simulink model "Fuel_Pump_V3_1_20201113_20KHz"  (R2019b)
settings: configuration reference "Configuration" (kept outside this file)
PreLoadFcn:
  | RTWConfigurationCB('preloadfcn', bdroot);
values from neighbouring files (symbols this model uses):
  MotorPara_Base_Frq = 666.0    [fuel_pump_V3_1_20201113_20kHz.sldd]
  MotorPara_Base_I = 50.0    [fuel_pump_V3_1_20201113_20kHz.sldd]
  MotorPara_Base_RPM = 12000.0    [fuel_pump_V3_1_20201113_20kHz.sldd]
  MotorPara_Base_V = 28.0    [fuel_pump_V3_1_20201113_20kHz.sldd]
  MotorPara_Ld = 1.287E-5    [fuel_pump_V3_1_20201113_20kHz.sldd]
  MotorPara_Lq = 2.052E-5    [fuel_pump_V3_1_20201113_20kHz.sldd]
  MotorPara_Ls = 8.3475E-5    [fuel_pump_V3_1_20201113_20kHz.sldd]
  MotorPara_P = 4.0    [fuel_pump_V3_1_20201113_20kHz.sldd]
  MotorPara_Rs = 0.01638    [fuel_pump_V3_1_20201113_20kHz.sldd]
  TPBRD_HALF = 1875.0    [fuel_pump_V3_1_20201113_20kHz.sldd]
  Ts_1kHz = 0.001    [fuel_pump_V3_1_20201113_20kHz.sldd]
  Ts_200Hz = 0.005    [fuel_pump_V3_1_20201113_20kHz.sldd]
  Ts_20KHz = 5.0E-5    [fuel_pump_V3_1_20201113_20kHz.sldd]
  Ts_40Hz = 0.025    [fuel_pump_V3_1_20201113_20kHz.sldd]
  Ts_50Hz = 0.02    [fuel_pump_V3_1_20201113_20kHz.sldd]
undefined symbols (not defined in the file or in its folder): DiscIntNeverNeededParam, Down, Up
libraries: c280xlib x22, c2833xlib x6, c2837xDlib x4, c28xdmclib x4, etargetslib x4, dspstat3 x2, c2000lib x1, idelinklib_common x1
(part 2 of 4)

== system Fuel_Pump_V3_1_20201113_20KHz/SCI_TX ==
  1-D Lookup Table2 : Lookup_n-D  Commented=on  NumberOfTableDimensions=1  BreakpointsForDimension1=[0,9.84,53.12,85.06,128.14,168.25,208.63,249.25,290.69,331.14,368.31]  Table=[0,-1000,-2000,-3000,-4000,-5000,-6000,-7000,-8000,-9000,-10000]  InternalRulePriority=Speed  RndMeth=Simplest  InputSameDT=on
  Data Store Read13 : DataStoreRead  Commented=on  DataStoreName=WFm
  Data Store Write : DataStoreWrite  Commented=on  DataStoreName=nDem
  FPM : Subsystem
  MATLAB Function49 : MATLAB Function  Commented=on  TreatAsAtomicUnit=on
  SCI Receive2 : c280xlib/SCI Receive  Commented=on  sciModule=A  dataHead='~~'  dataTail=''  dataType=uint8  dataDim=10  initValue=0  errOption=Output custom value  errValue=[255,0,0,0,0,0,0,0,0,255]  sampleTime=Ts_SCI  outputStatus=off  postInterrupt=off  numFifo=10
      settings: SourceProductName=Embedded Coder Support Package for Texas Instruments C2000 Processors  SourceProductBaseCode=TIC2000
  SCI Transmit : c280xlib/SCI Transmit  sciModule=A  dataHead=''  dataTail=''  postInterrupt=off  numFifo=1
      settings: SourceProductName=Embedded Coder Support Package for Texas Instruments C2000 Processors
  SCI_TX : Subsystem
  Saturation : Saturate  Commented=on  UpperLimit=0  LowerLimit=-12000
  wires:
  Data Store Read13/1 -> 1-D Lookup Table2/1
  1-D Lookup Table2/1 -> Saturation/1
  Saturation/1 -> Data Store Write/1
  SCI Receive2/1 -> MATLAB Function49/1(Data_SCI)
  SCI_TX/1(SCI_DATA) -> SCI Transmit/1

== system Fuel_Pump_V3_1_20201113_20KHz/Set_nDem ==
  Data Store Read1 : DataStoreRead  DataStoreName=n_Step
  Data Store Read2 : DataStoreRead  DataStoreName=nDem
  Data Store Read3 : DataStoreRead  Commented=on  DataStoreName=LWF_Step
  Data Store Read4 : DataStoreRead  Commented=on  DataStoreName=LWFDem
  Data Store Write1 : DataStoreWrite  DataStoreName=nDem_PI
  Data Store Write2 : DataStoreWrite  Commented=on  DataStoreName=Set_Speed
  Data Store Write3 : DataStoreWrite  Commented=on  DataStoreName=SMO_KP
  Data Store Write4 : DataStoreWrite  Commented=on  DataStoreName=SMO_KI
  Data Store Write5 : DataStoreWrite  DataStoreName=SMO_Filter
  Gain : Gain  Gain=1/MotorPara_Base_RPM
  Gain1 : Gain  Gain=MotorPara_Base_RPM
  Gain2 : Gain  Commented=on  Gain=13/3  OutDataTypeStr=Inherit: Inherit via back propagation
  Gain3 : Gain  Commented=on  Gain=15000  OutDataTypeStr=Inherit: Inherit via back propagation
  Gain4 : Gain  Commented=on  Gain=5*2*pi/60*4
  Gain5 : Gain  Commented=on  Gain=2
  Gain6 : Gain  Gain=10
  Gain7 : Gain  Gain=-1
  MATLAB Function1 : MATLAB Function  TreatAsAtomicUnit=on
  MATLAB Function2 : MATLAB Function  Commented=on  TreatAsAtomicUnit=on
  Square : Math  Commented=on  Operator=square  SignedPower=off  SaturateOnIntegerOverflow=on
  wires:
  Data Store Read2/1 -> Gain/1
  MATLAB Function1/1(Set_Point) -> Gain1/1
  Data Store Read1/1 -> MATLAB Function1/2(Step)
  Data Store Read4/1 -> Gain2/1
  Data Store Read3/1 -> MATLAB Function2/2(Step)
  Gain3/1 -> Data Store Write2/1
  Gain2/1 -> MATLAB Function2/1(Target)
  MATLAB Function2/1(Set_Point) -> Gain3/1
  Gain/1 -> MATLAB Function1/1(Target)
  Gain1/1 -> Gain7/1, Data Store Write1/1
  Gain4/1 -> Square/1, Gain5/1
  Gain5/1 -> Data Store Write3/1
  Square/1 -> Data Store Write4/1
  Gain6/1 -> Data Store Write5/1
  Gain7/1 -> Gain6/1, Gain4/1

== system Fuel_Pump_V3_1_20201113_20KHz/System Initialize ==

== system Fuel_Pump_V3_1_20201113_20KHz/IIC_Interrupt /Subsystem ==
  function : TriggerPort  TriggerType=function-call  VariantControl=Variant
  Data Store Write2 : DataStoreWrite  DataStoreName=TEMP_MOT1
  Demux : Demux  Outputs=2
  I2C Receive : c280xlib/I2C Receive  Priority=1  selectModule=I2C_A  addrFormat=7-Bit addressing  saSource=Specify via dialog  SAR=64  bitCount=8  dataLength=2  initValue=0  NACK=off  STP=on  STR=off  sampleTime=-1  dataType=uint8
      settings: SourceProductName=Embedded Coder Support Package for Texas Instruments C2000 Processors  SourceProductBaseCode=TIC2000
  Temp_conv : MATLAB Function  TreatAsAtomicUnit=on
  wires:
  Temp_conv/1(y) -> Data Store Write2/1
  I2C Receive/1 -> Demux/1
  Demux/2 -> Temp_conv/2(u2)
  Demux/1 -> Temp_conv/1(u1)

== system Fuel_Pump_V3_1_20201113_20KHz/IIC_Interrupt /Subsystem1 ==
  function : TriggerPort  TriggerType=function-call  VariantControl=Variant
  Data Store Write2 : DataStoreWrite  DataStoreName=TEMP_MOT2
  Demux : Demux  Outputs=2
  I2C Receive : c280xlib/I2C Receive  Priority=1  selectModule=I2C_A  addrFormat=7-Bit addressing  saSource=Specify via dialog  SAR=65  bitCount=8  dataLength=2  initValue=0  NACK=off  STP=on  STR=off  sampleTime=-1  dataType=uint8
      settings: SourceProductName=Embedded Coder Support Package for Texas Instruments C2000 Processors  SourceProductBaseCode=TIC2000
  Temp_conv : MATLAB Function  TreatAsAtomicUnit=on
  wires:
  Demux/1 -> Temp_conv/1(u1)
  Demux/2 -> Temp_conv/2(u2)
  I2C Receive/1 -> Demux/1
  Temp_conv/1(y) -> Data Store Write2/1

== system Fuel_Pump_V3_1_20201113_20KHz/IIC_PT1000/Subsystem4 ==
  function : TriggerPort  TriggerType=function-call  VariantControl=Variant
  Constant : Constant  Value=16  OutDataTypeStr=uint8  SampleTime=-1
  I2C Transmit : c280xlib/I2C Transmit  selectModule=I2C_A  addrFormat=7-Bit addressing  saSource=Specify via dialog  SAR=64  bitCount=8  STP=off  RM=off  STR=off
      settings: SourceProductName=Embedded Coder Support Package for Texas Instruments C2000 Processors  SourceProductBaseCode=TIC2000
  wires:
  Constant/1 -> I2C Transmit/1

== system Fuel_Pump_V3_1_20201113_20KHz/IIC_PT1000/Subsystem5 ==
  function : TriggerPort  TriggerType=function-call  VariantControl=Variant
  Constant : Constant  Value=16  OutDataTypeStr=uint8  SampleTime=-1
  I2C Transmit : c280xlib/I2C Transmit  selectModule=I2C_A  addrFormat=7-Bit addressing  saSource=Specify via dialog  SAR=65  bitCount=8  STP=off  RM=off  STR=off
      settings: SourceProductName=Embedded Coder Support Package for Texas Instruments C2000 Processors  SourceProductBaseCode=TIC2000
  wires:
  Constant/1 -> I2C Transmit/1

== system Fuel_Pump_V3_1_20201113_20KHz/Motor_Control/Initial Case ==
  Action Port : ActionPort  ActionPortLabel=case [ 0 ]:

== system Fuel_Pump_V3_1_20201113_20KHz/Motor_Control/Interrupt_Count ==
  Add : Sum
  Constant : Constant  OutDataTypeStr=uint16  SampleTime=-1
  Constant1 : Constant  Value=0.00005  OutDataTypeStr=single  SampleTime=-1
  Product : Product  OutDataTypeStr=uint8
  Saturation : Saturate  UpperLimit=40000  LowerLimit=0
  Unit Delay : UnitDelay  SampleTime=-1  HasFrameUpgradeWarning=on
  Out1 : Outport
  wires:
  Product/1 -> Out1/1
  Unit Delay/1 -> Add/2
  Add/1 -> Saturation/1
  Saturation/1 -> Product/2, Unit Delay/1
  Constant1/1 -> Product/1
  Constant/1 -> Add/1

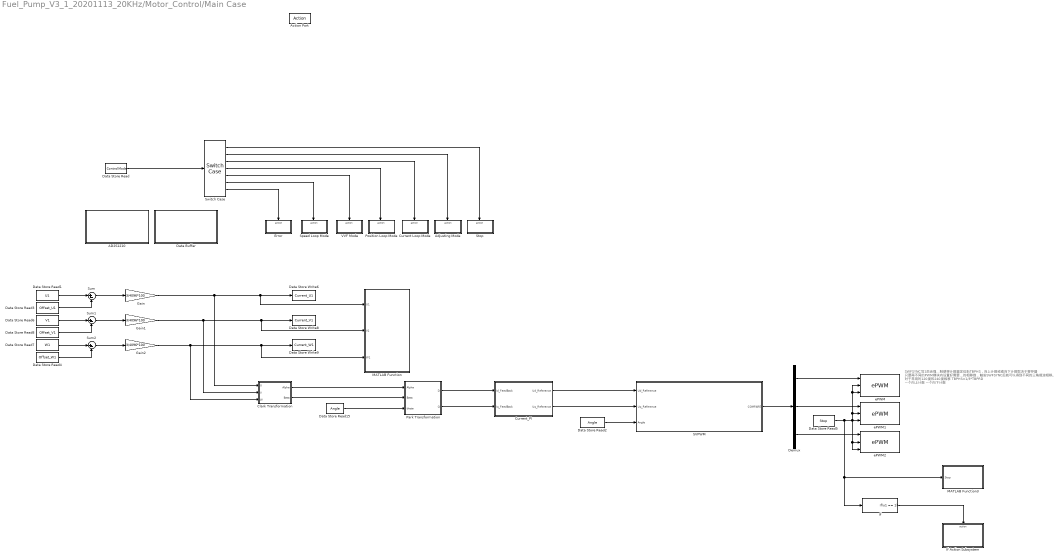
== system Fuel_Pump_V3_1_20201113_20KHz/Motor_Control/Main Case  ==
  note: SWFSYNC写1后会强制使得计数器定位到TBPHS，向上计数或者向下计数取决于寄存器
      |
      | 只要再不同的PWM模块内设置好需要的相移数，触发SWFSYNC后就可以得到不同的三角载波相移。
      |
      | 对于常用的120度和240度相移
      | TBPHS=1/3*TBPRD 一个向上计数 一个向下计数
  Action Port : ActionPort  ActionPortLabel=case [ 2 ]:
  AD2S1210 : Subsystem  Priority=30  TreatAsAtomicUnit=on
  Adjusting Mode : Subsystem  TreatAsAtomicUnit=on
  Clark Transformation : Subsystem
  Current Loop Mode : Subsystem  TreatAsAtomicUnit=on
  Current_PI : Subsystem  TreatAsAtomicUnit=on
      settings: RTWSystemCode=Inline
  "Data Buffer " : Subsystem
  Data Store Read : DataStoreRead  Priority=40  DataStoreName=ControlMode
  Data Store Read1 : DataStoreRead  DataStoreName=U1
  Data Store Read15 : DataStoreRead  Priority=62  DataStoreName=Angle
  Data Store Read2 : DataStoreRead  DataStoreName=Angle
  Data Store Read3 : DataStoreRead  DataStoreName=Offset_U1
  Data Store Read4 : DataStoreRead  DataStoreName=Offset_W1
  Data Store Read5 : DataStoreRead  DataStoreName=Stop
  Data Store Read6 : DataStoreRead  DataStoreName=V1
  Data Store Read7 : DataStoreRead  DataStoreName=W1
  Data Store Read8 : DataStoreRead  DataStoreName=Offset_V1
  Data Store Write6 : DataStoreWrite  DataStoreName=Current_U1
  Data Store Write8 : DataStoreWrite  DataStoreName=Current_V1
  Data Store Write9 : DataStoreWrite  DataStoreName=Current_W1
  Demux : Demux  Outputs=3
  Error : Subsystem  TreatAsAtomicUnit=on
  Gain : Gain  Gain=3/4096*100  OutDataTypeStr=single
  Gain1 : Gain  Gain=3/4096*100  OutDataTypeStr=single
  Gain2 : Gain  Gain=3/4096*100  OutDataTypeStr=single
  If : If  IfExpression=u1 == 1  ShowElse=off
  If Action Subsystem : Subsystem  TreatAsAtomicUnit=on
  MATLAB Function : MATLAB Function  TreatAsAtomicUnit=on
  MATLAB Function3 : MATLAB Function  TreatAsAtomicUnit=on
  Park Transformation : Subsystem
  Position Loop Mode : Subsystem  TreatAsAtomicUnit=on
  SVPWM : Subsystem  TreatAsAtomicUnit=on
      settings: RTWSystemCode=Inline
  Speed Loop Mode : Subsystem  TreatAsAtomicUnit=on
  Stop : Subsystem  TreatAsAtomicUnit=on
  Sum : Sum  Inputs=|+-  AccumDataTypeStr=int16  OutDataTypeStr=int16  InputSameDT=on
  Sum1 : Sum  Inputs=|+-  AccumDataTypeStr=int16  OutDataTypeStr=int16  InputSameDT=on
  Sum2 : Sum  Inputs=|+-  AccumDataTypeStr=int16  OutDataTypeStr=int16  InputSameDT=on
  Switch Case : SwitchCase  CaseConditions={0,1,2,3,4,5}
  VVF Mode : Subsystem  TreatAsAtomicUnit=on
  ePWM : c280xlib/ePWM  checkMode=off  useModule=ePWM1  periodUnits=Clock cycles  timerSource=Specify via dialog  timerPeriod_clk=TPBRD  timerPeriod_sec=0.0001  tbshadow=Counter equals to zero  countingMode=Up-Down  phaseActiveEnable=Set counter to phase value specified via dialog  phaseDirection=Count down after sync  phaseActive=0  synchronizationEnable=off  synchronizationOption=Counter equals to zero (CTR=Zero)  clockPrescale=1  HSclockPrescale=1  ePWMxAStatus=on  CMPAUnits=Clock cycles  CMPASource=Input port  CMPAValue_per=50  CMPAValue_clk=0  enCMPAshadow=Counter equals to zero  ePWMxAactionLogic1=Do nothing  ePWMxAactionLogic2=Do nothing  ePWMxAactionLogic3=Set  ePWMxAactionLogic4=Clear  ePWMxAactionLogic5=Do nothing  ePWMxAactionLogic6=Do nothing  ePWMxALoadMode=Load on counter equals to zero (CTR=Zero)  ePWMxACSFenable=on  ePWMxACSFvalue=Forcing disable  ePWMxASFreload=Immediate  enHRPWM=off  HRPWM_LoadMode=Counter equals to zero (CTR=ZERO)  HRPWM_CTLMode=Phase control mode  HRPWM_EDGMode=Both edge  enSFO=on  ePWMxBStatus=on  CMPBUnits=Clock cycles  CMPBSource=Specify via dialog  CMPBValue_per=50  CMPBValue_clk=0  enCMPBshadow=Counter equals to zero  ePWMxBactionLogic1=Do nothing  ePWMxBactionLogic2=Do nothing  ePWMxBactionLogic3=Set  ePWMxBactionLogic4=Clear  ePWMxBactionLogic5=Do nothing  ePWMxBactionLogic6=Do nothing  ePWMxBLoadMode=Load on counter equals to zero (CTR=Zero)  ePWMxBCSFenable=on  ePWMxBCSFvalue=Forcing disable  ePWMxBSFreload=Immediate  enableDBePWMxA=on  enableDBePWMxB=on  DBpolarity=Active high (AH)  DBedgeDelay=Negative  DBSource_ePWMxA=ePWMxA  DBSource_ePWMxB=ePWMxA  DBperiodSource=Specify via dialog  REDperiod=TDEAD  FEDperiod=TDEAD  adcstartModuleA=on  adcrequestEventA=First event  adcstartEventA=Counter equals to zero (CTR=Zero)  adcstartModuleB=off  adcrequestEventB=First event  adcstartEventB=Counter equals to zero (CTR=Zero)  intEn=off  intPrd=First event  intSel=Counter equals to zero (CTR=Zero)  chopperEnable=off  chopperFrequency=1  chopperFirstwidth=1  chopperDuty=12.5%  tripZonesource=Specify via dialog  tzselOSHT1=off  tzselOSHT2=off  tzselOSHT3=off  tzselOSHT4=off  tzselOSHT5=off  tzselOSHT6=off  tzselCBC1=off  tzselCBC2=off  tzselCBC3=off  tzselCBC4=off  tzselCBC5=off  tzselCBC6=off  enTzOstIntr=off  enTzCbcIntr=off  ePWMxAforced=No action  ePWMxBforced=No action  timerPeriod=-1  ePWMxAValue=0  ePWMxBValue=0  tripZoneoption=One-shot trip (OSHT)
      settings: SourceProductName=Embedded Coder Support Package for Texas Instruments C2000 Processors  SourceProductBaseCode=TIC2000
  ePWM1 : c280xlib/ePWM  checkMode=off  useModule=ePWM2  periodUnits=Clock cycles  timerSource=Specify via dialog  timerPeriod_clk=TPBRD  timerPeriod_sec=0.0001  tbshadow=Counter equals to zero  countingMode=Up-Down  phaseActiveEnable=Set counter to phase value specified via dialog  phaseDirection=Count down after sync  phaseActive=0  synchronizationEnable=off  synchronizationOption=Counter equals to zero (CTR=Zero)  clockPrescale=1  HSclockPrescale=1  ePWMxAStatus=on  CMPAUnits=Clock cycles  CMPASource=Input port  CMPAValue_per=50  CMPAValue_clk=0  enCMPAshadow=Counter equals to zero  ePWMxAactionLogic1=Do nothing  ePWMxAactionLogic2=Do nothing  ePWMxAactionLogic3=Set  ePWMxAactionLogic4=Clear  ePWMxAactionLogic5=Do nothing  ePWMxAactionLogic6=Do nothing  ePWMxALoadMode=Load on counter equals to zero (CTR=Zero)  ePWMxACSFenable=on  ePWMxACSFvalue=Forcing disable  ePWMxASFreload=Immediate  enHRPWM=off  HRPWM_LoadMode=Counter equals to zero (CTR=ZERO)  HRPWM_CTLMode=Phase control mode  HRPWM_EDGMode=Both edge  enSFO=on  ePWMxBStatus=on  CMPBUnits=Clock cycles  CMPBSource=Specify via dialog  CMPBValue_per=50  CMPBValue_clk=0  enCMPBshadow=Counter equals to zero  ePWMxBactionLogic1=Do nothing  ePWMxBactionLogic2=Do nothing  ePWMxBactionLogic3=Set  ePWMxBactionLogic4=Clear  ePWMxBactionLogic5=Do nothing  ePWMxBactionLogic6=Do nothing  ePWMxBLoadMode=Load on counter equals to zero (CTR=Zero)  ePWMxBCSFenable=on  ePWMxBCSFvalue=Forcing disable  ePWMxBSFreload=Immediate  enableDBePWMxA=on  enableDBePWMxB=on  DBpolarity=Active high (AH)  DBedgeDelay=Positive  DBSource_ePWMxA=ePWMxA  DBSource_ePWMxB=ePWMxA  DBperiodSource=Specify via dialog  REDperiod=TDEAD  FEDperiod=TDEAD  adcstartModuleA=off  adcrequestEventA=First event  adcstartEventA=Counter equals to period (CTR=PRD)  adcstartModuleB=off  adcrequestEventB=First event  adcstartEventB=Counter equals to zero (CTR=Zero)  intEn=off  intPrd=First event  intSel=Counter equals to zero (CTR=Zero)  chopperEnable=off  chopperFrequency=1  chopperFirstwidth=1  chopperDuty=12.5%  tripZonesource=Specify via dialog  tzselOSHT1=off  tzselOSHT2=off  tzselOSHT3=off  tzselOSHT4=off  tzselOSHT5=off  tzselOSHT6=off  tzselCBC1=off  tzselCBC2=off  tzselCBC3=off  tzselCBC4=off  tzselCBC5=off  tzselCBC6=off  enTzOstIntr=off  enTzCbcIntr=off  ePWMxAforced=No action  ePWMxBforced=No action  timerPeriod=-1  ePWMxAValue=0  ePWMxBValue=0  tripZoneoption=One-shot trip (OSHT)
      settings: SourceProductName=Embedded Coder Support Package for Texas Instruments C2000 Processors  SourceProductBaseCode=TIC2000
  ePWM2 : c280xlib/ePWM  checkMode=off  useModule=ePWM3  periodUnits=Clock cycles  timerSource=Specify via dialog  timerPeriod_clk=TPBRD  timerPeriod_sec=0.0001  tbshadow=Counter equals to zero  countingMode=Up-Down  phaseActiveEnable=Set counter to phase value specified via dialog  phaseDirection=Count down after sync  phaseActive=0  synchronizationEnable=off  synchronizationOption=Counter equals to zero (CTR=Zero)  clockPrescale=1  HSclockPrescale=1  ePWMxAStatus=on  CMPAUnits=Clock cycles  CMPASource=Input port  CMPAValue_per=50  CMPAValue_clk=0  enCMPAshadow=Counter equals to zero  ePWMxAactionLogic1=Do nothing  ePWMxAactionLogic2=Do nothing  ePWMxAactionLogic3=Set  ePWMxAactionLogic4=Clear  ePWMxAactionLogic5=Do nothing  ePWMxAactionLogic6=Do nothing  ePWMxALoadMode=Load on counter equals to zero (CTR=Zero)  ePWMxACSFenable=on  ePWMxACSFvalue=Forcing disable  ePWMxASFreload=Immediate  enHRPWM=off  HRPWM_LoadMode=Counter equals to zero (CTR=ZERO)  HRPWM_CTLMode=Phase control mode  HRPWM_EDGMode=Both edge  enSFO=on  ePWMxBStatus=on  CMPBUnits=Clock cycles  CMPBSource=Specify via dialog  CMPBValue_per=50  CMPBValue_clk=0  enCMPBshadow=Counter equals to zero  ePWMxBactionLogic1=Do nothing  ePWMxBactionLogic2=Do nothing  ePWMxBactionLogic3=Set  ePWMxBactionLogic4=Clear  ePWMxBactionLogic5=Do nothing  ePWMxBactionLogic6=Do nothing  ePWMxBLoadMode=Load on counter equals to zero (CTR=Zero)  ePWMxBCSFenable=on  ePWMxBCSFvalue=Forcing disable  ePWMxBSFreload=Immediate  enableDBePWMxA=on  enableDBePWMxB=on  DBpolarity=Active high (AH)  DBedgeDelay=Positive  DBSource_ePWMxA=ePWMxA  DBSource_ePWMxB=ePWMxA  DBperiodSource=Specify via dialog  REDperiod=TDEAD  FEDperiod=TDEAD  adcstartModuleA=off  adcrequestEventA=First event  adcstartEventA=Counter equals to period (CTR=PRD)  adcstartModuleB=off  adcrequestEventB=First event  adcstartEventB=Counter equals to zero (CTR=Zero)  intEn=off  intPrd=First event  intSel=Counter equals to zero (CTR=Zero)  chopperEnable=off  chopperFrequency=1  chopperFirstwidth=1  chopperDuty=12.5%  tripZonesource=Specify via dialog  tzselOSHT1=off  tzselOSHT2=off  tzselOSHT3=off  tzselOSHT4=off  tzselOSHT5=off  tzselOSHT6=off  tzselCBC1=off  tzselCBC2=off  tzselCBC3=off  tzselCBC4=off  tzselCBC5=off  tzselCBC6=off  enTzOstIntr=off  enTzCbcIntr=off  ePWMxAforced=No action  ePWMxBforced=No action  timerPeriod=-1  ePWMxAValue=0  ePWMxBValue=0  tripZoneoption=One-shot trip (OSHT)
      settings: SourceProductName=Embedded Coder Support Package for Texas Instruments C2000 Processors  SourceProductBaseCode=TIC2000
  wires:
  Switch Case/4 -> Position Loop Mode/Action
  Switch Case/7 -> Error/Action
  Clark Transformation/1(Alpha) -> Park Transformation/1(Alpha)
  Current_PI/2(Uq_Reference) -> SVPWM/2(Uq_Reference)
  Current_PI/1(Ud_Reference) -> SVPWM/1(Ud_Reference)
  Park Transformation/1(D) -> Current_PI/1(Id_FeedBack)
  Park Transformation/2(Q) -> Current_PI/2(Iq_FeedBack)
  SVPWM/1(COMPARE) -> Demux/1
  Data Store Read2/1 -> SVPWM/3(Angle)
  Data Store Read5/1 -> If/1, MATLAB Function3/1(Stop), ePWM1/3, ePWM2/2, ePWM2/3, ePWM1/2, ePWM/2, ePWM/3
  Switch Case/5 -> VVF Mode/Action
  Data Store Read3/1 -> Sum/2
  Data Store Read8/1 -> Sum1/2
  Sum/1 -> Gain/1
  Data Store Read4/1 -> Sum2/2
  Data Store Read7/1 -> Sum2/1
  Data Store Read6/1 -> Sum1/1
  Data Store Read1/1 -> Sum/1
  Sum1/1 -> Gain1/1
  Sum2/1 -> Gain2/1
  Clark Transformation/2(Beta) -> Park Transformation/2(Beta)
  Data Store Read15/1 -> Park Transformation/3(theta)
  Gain/1 -> Clark Transformation/1(U), Data Store Write6/1, MATLAB Function/1(U1)
  Gain1/1 -> Clark Transformation/2(V), Data Store Write8/1, MATLAB Function/2(V1)
  Gain2/1 -> Clark Transformation/3(W), Data Store Write9/1, MATLAB Function/3(W1)
  Demux/1 -> ePWM/1
  Demux/2 -> ePWM1/1
  Demux/3 -> ePWM2/1
  Data Store Read/1 -> Switch Case/1
  Switch Case/6 -> Speed Loop Mode/Action
  Switch Case/3 -> Current Loop Mode/Action
  Switch Case/2 -> Adjusting Mode/Action
  Switch Case/1 -> Stop/Action
  If/1 -> If Action Subsystem/Action

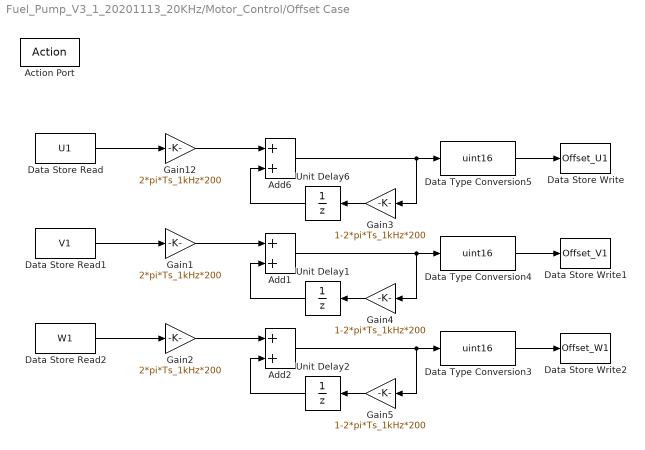
== system Fuel_Pump_V3_1_20201113_20KHz/Motor_Control/Offset Case  ==
  Action Port : ActionPort  ActionPortLabel=case [ 1 ]:
  Add1 : Sum  OutDataTypeStr=Inherit: Inherit via back propagation
  Add2 : Sum  OutDataTypeStr=Inherit: Inherit via back propagation
  Add6 : Sum  OutDataTypeStr=Inherit: Inherit via back propagation
  Data Store Read : DataStoreRead  DataStoreName=U1
  Data Store Read1 : DataStoreRead  DataStoreName=V1
  Data Store Read2 : DataStoreRead  DataStoreName=W1
  Data Store Write : DataStoreWrite  DataStoreName=Offset_U1
  Data Store Write1 : DataStoreWrite  DataStoreName=Offset_V1
  Data Store Write2 : DataStoreWrite  DataStoreName=Offset_W1
  Data Type Conversion3 : DataTypeConversion  OutDataTypeStr=uint16
  Data Type Conversion4 : DataTypeConversion  OutDataTypeStr=uint16
  Data Type Conversion5 : DataTypeConversion  OutDataTypeStr=uint16
  Gain1 : Gain  Gain=2*pi*Ts_1kHz*200  ParamDataTypeStr=double  OutDataTypeStr=single
  Gain12 : Gain  Gain=2*pi*Ts_1kHz*200  ParamDataTypeStr=double  OutDataTypeStr=single
  Gain2 : Gain  Gain=2*pi*Ts_1kHz*200  ParamDataTypeStr=double  OutDataTypeStr=single
  Gain3 : Gain  Gain=1-2*pi*Ts_1kHz*200  OutDataTypeStr=Inherit: Inherit via back propagation
  Gain4 : Gain  Gain=1-2*pi*Ts_1kHz*200  OutDataTypeStr=Inherit: Inherit via back propagation
  Gain5 : Gain  Gain=1-2*pi*Ts_1kHz*200  OutDataTypeStr=Inherit: Inherit via back propagation
  Unit Delay1 : UnitDelay  SampleTime=-1  HasFrameUpgradeWarning=on
  Unit Delay2 : UnitDelay  SampleTime=-1  HasFrameUpgradeWarning=on
  Unit Delay6 : UnitDelay  SampleTime=-1  HasFrameUpgradeWarning=on
  wires:
  Add6/1 -> Data Type Conversion5/1, Gain3/1
  Data Store Read/1 -> Gain12/1
  Gain12/1 -> Add6/1
  Gain3/1 -> Unit Delay6/1
  Unit Delay6/1 -> Add6/2
  Data Type Conversion3/1 -> Data Store Write2/1
  Data Type Conversion4/1 -> Data Store Write1/1
  Data Type Conversion5/1 -> Data Store Write/1
  Unit Delay1/1 -> Add1/2
  Gain4/1 -> Unit Delay1/1
  Gain1/1 -> Add1/1
  Data Store Read1/1 -> Gain1/1
  Add1/1 -> Gain4/1, Data Type Conversion4/1
  Add2/1 -> Gain5/1, Data Type Conversion3/1
  Gain2/1 -> Add2/1
  Gain5/1 -> Unit Delay2/1
  Unit Delay2/1 -> Add2/2
  Data Store Read2/1 -> Gain2/1

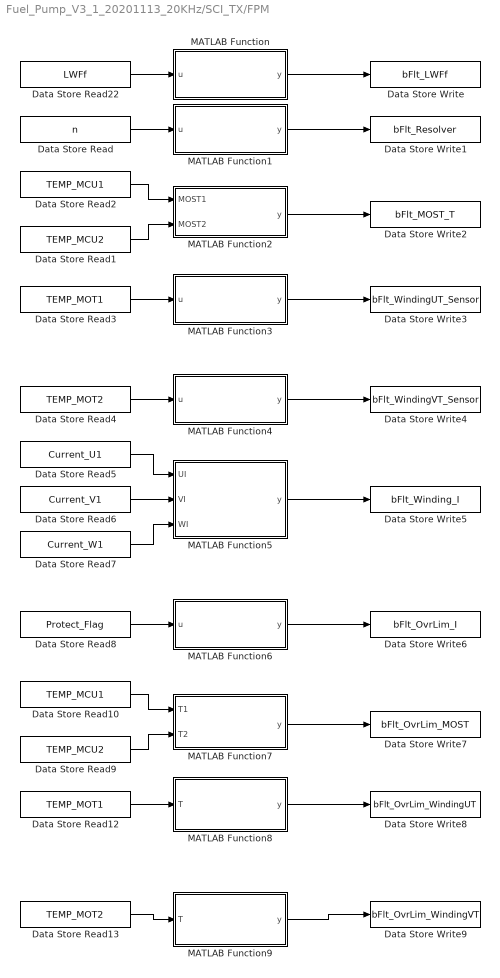
== system Fuel_Pump_V3_1_20201113_20KHz/SCI_TX/FPM ==
  Data Store Read : DataStoreRead  DataStoreName=n  SampleTime=Ts_40Hz
  Data Store Read1 : DataStoreRead  DataStoreName=TEMP_MCU2  SampleTime=Ts_40Hz
  Data Store Read10 : DataStoreRead  DataStoreName=TEMP_MCU1  SampleTime=Ts_40Hz
  Data Store Read12 : DataStoreRead  DataStoreName=TEMP_MOT1  SampleTime=Ts_40Hz
  Data Store Read13 : DataStoreRead  DataStoreName=TEMP_MOT2  SampleTime=Ts_40Hz
  Data Store Read2 : DataStoreRead  DataStoreName=TEMP_MCU1  SampleTime=Ts_40Hz
  Data Store Read22 : DataStoreRead  DataStoreName=LWFf  SampleTime=Ts_40Hz
  Data Store Read3 : DataStoreRead  DataStoreName=TEMP_MOT1  SampleTime=Ts_40Hz
  Data Store Read4 : DataStoreRead  DataStoreName=TEMP_MOT2  SampleTime=Ts_40Hz
  Data Store Read5 : DataStoreRead  DataStoreName=Current_U1  SampleTime=Ts_40Hz
  Data Store Read6 : DataStoreRead  DataStoreName=Current_V1  SampleTime=Ts_40Hz
  Data Store Read7 : DataStoreRead  DataStoreName=Current_W1  SampleTime=Ts_40Hz
  Data Store Read8 : DataStoreRead  DataStoreName=Protect_Flag  SampleTime=Ts_40Hz
  Data Store Read9 : DataStoreRead  DataStoreName=TEMP_MCU2  SampleTime=Ts_40Hz
  Data Store Write : DataStoreWrite  DataStoreName=bFlt_LWFf
  Data Store Write1 : DataStoreWrite  DataStoreName=bFlt_Resolver
  Data Store Write2 : DataStoreWrite  DataStoreName=bFlt_MOST_T
  Data Store Write3 : DataStoreWrite  DataStoreName=bFlt_WindingUT_Sensor
  Data Store Write4 : DataStoreWrite  DataStoreName=bFlt_WindingVT_Sensor
  Data Store Write5 : DataStoreWrite  DataStoreName=bFlt_Winding_I
  Data Store Write6 : DataStoreWrite  DataStoreName=bFlt_OvrLim_I
  Data Store Write7 : DataStoreWrite  DataStoreName=bFlt_OvrLim_MOST
  Data Store Write8 : DataStoreWrite  DataStoreName=bFlt_OvrLim_WindingUT
  Data Store Write9 : DataStoreWrite  DataStoreName=bFlt_OvrLim_WindingVT
  MATLAB Function : MATLAB Function  TreatAsAtomicUnit=on
  MATLAB Function1 : MATLAB Function  TreatAsAtomicUnit=on
  MATLAB Function2 : MATLAB Function  TreatAsAtomicUnit=on
  MATLAB Function3 : MATLAB Function  TreatAsAtomicUnit=on
  MATLAB Function4 : MATLAB Function  TreatAsAtomicUnit=on
  MATLAB Function5 : MATLAB Function  TreatAsAtomicUnit=on
  MATLAB Function6 : MATLAB Function  TreatAsAtomicUnit=on
  MATLAB Function7 : MATLAB Function  TreatAsAtomicUnit=on
  MATLAB Function8 : MATLAB Function  TreatAsAtomicUnit=on
  MATLAB Function9 : MATLAB Function  TreatAsAtomicUnit=on
  wires:
  Data Store Read22/1 -> MATLAB Function/1(u)
  MATLAB Function/1(y) -> Data Store Write/1
  MATLAB Function1/1(y) -> Data Store Write1/1
  Data Store Read/1 -> MATLAB Function1/1(u)
  Data Store Read2/1 -> MATLAB Function2/1(MOST1)
  MATLAB Function2/1(y) -> Data Store Write2/1
  Data Store Read1/1 -> MATLAB Function2/2(MOST2)
  Data Store Read3/1 -> MATLAB Function3/1(u)
  MATLAB Function3/1(y) -> Data Store Write3/1
  MATLAB Function4/1(y) -> Data Store Write4/1
  Data Store Read4/1 -> MATLAB Function4/1(u)
  Data Store Read5/1 -> MATLAB Function5/1(UI)
  Data Store Read6/1 -> MATLAB Function5/2(VI)
  Data Store Read7/1 -> MATLAB Function5/3(WI)
  MATLAB Function5/1(y) -> Data Store Write5/1
  Data Store Read8/1 -> MATLAB Function6/1(u)
  MATLAB Function6/1(y) -> Data Store Write6/1
  Data Store Read10/1 -> MATLAB Function7/1(T1)
  Data Store Read9/1 -> MATLAB Function7/2(T2)
  MATLAB Function7/1(y) -> Data Store Write7/1
  Data Store Read12/1 -> MATLAB Function8/1(T)
  MATLAB Function8/1(y) -> Data Store Write8/1
  MATLAB Function9/1(y) -> Data Store Write9/1
  Data Store Read13/1 -> MATLAB Function9/1(T)

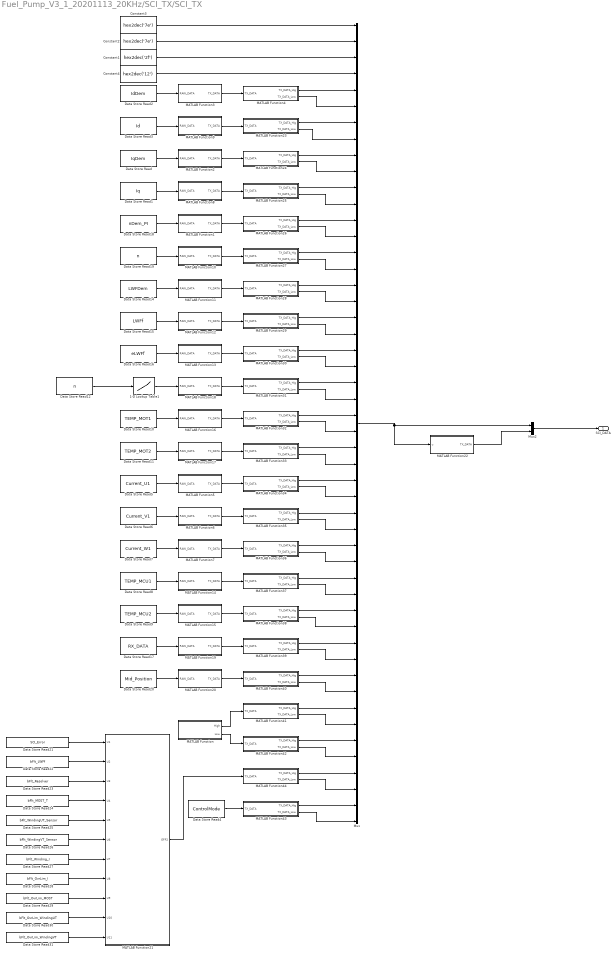
== system Fuel_Pump_V3_1_20201113_20KHz/SCI_TX/SCI_TX ==
  1-D Lookup Table1 : Lookup_n-D  NumberOfTableDimensions=1  BreakpointsForDimension1=[-10000,-9000,-8000,-7000,-6000,-5000,-4000,-3000,-2000,-1000,0]  Table=[368.31,331.14,290.69,249.25,208.63,168.25,128.14,85.06,53.12,9.84,0]  InternalRulePriority=Speed  RndMeth=Simplest  InputSameDT=on
  Constant1 : Constant  Priority=100  Value=hex2dec('2f')  OutDataTypeStr=uint8  SampleTime=Ts_40Hz
  Constant2 : Constant  Priority=100  Value=hex2dec('7e')  OutDataTypeStr=uint8  SampleTime=Ts_40Hz
  Constant3 : Constant  Priority=100  Value=hex2dec('7e')  OutDataTypeStr=uint8  SampleTime=Ts_40Hz
  Constant4 : Constant  Priority=100  Value=hex2dec('12')  OutDataTypeStr=uint8  SampleTime=Ts_40Hz
  Data Store Read : DataStoreRead  DataStoreName=IqDem
  Data Store Read1 : DataStoreRead  DataStoreName=Iq
  Data Store Read10 : DataStoreRead  DataStoreName=TEMP_MOT1
  Data Store Read11 : DataStoreRead  DataStoreName=TEMP_MOT2
  Data Store Read12 : DataStoreRead  DataStoreName=n
  Data Store Read14 : DataStoreRead  DataStoreName=LWFDem
  Data Store Read15 : DataStoreRead  DataStoreName=LWFf
  Data Store Read16 : DataStoreRead  DataStoreName=eLWFf
  Data Store Read17 : DataStoreRead  DataStoreName=RX_DATA
  Data Store Read18 : DataStoreRead  DataStoreName=nDem_PI
  Data Store Read19 : DataStoreRead  DataStoreName=n
  Data Store Read2 : DataStoreRead  DataStoreName=IdDem
  Data Store Read20 : DataStoreRead  DataStoreName=Mid_Position
  Data Store Read21 : DataStoreRead  DataStoreName=SCI_Error  SampleTime=Ts_40Hz
  Data Store Read22 : DataStoreRead  DataStoreName=bFlt_LWFf
  Data Store Read23 : DataStoreRead  DataStoreName=bFlt_Resolver
  Data Store Read24 : DataStoreRead  DataStoreName=bFlt_MOST_T
  Data Store Read25 : DataStoreRead  DataStoreName=bFlt_WindingUT_Sensor
  Data Store Read26 : DataStoreRead  DataStoreName=bFlt_WindingVT_Sensor
  Data Store Read27 : DataStoreRead  DataStoreName=bFlt_Winding_I
  Data Store Read28 : DataStoreRead  DataStoreName=bFlt_OvrLim_I
  Data Store Read29 : DataStoreRead  DataStoreName=bFlt_OvrLim_MOST
  Data Store Read3 : DataStoreRead  DataStoreName=Id
  Data Store Read30 : DataStoreRead  DataStoreName=bFlt_OvrLim_WindingUT
  Data Store Read31 : DataStoreRead  DataStoreName=bFlt_OvrLim_WindingVT
  Data Store Read4 : DataStoreRead  DataStoreName=ControlMode
  Data Store Read5 : DataStoreRead  DataStoreName=Current_U1
  Data Store Read6 : DataStoreRead  DataStoreName=Current_V1
  Data Store Read7 : DataStoreRead  DataStoreName=Current_W1
  Data Store Read8 : DataStoreRead  DataStoreName=TEMP_MCU1
  Data Store Read9 : DataStoreRead  DataStoreName=TEMP_MCU2
  MATLAB Function : MATLAB Function  TreatAsAtomicUnit=on
  MATLAB Function1 : MATLAB Function  TreatAsAtomicUnit=on
  MATLAB Function10 : MATLAB Function  TreatAsAtomicUnit=on
  MATLAB Function11 : MATLAB Function  TreatAsAtomicUnit=on
  MATLAB Function12 : MATLAB Function  TreatAsAtomicUnit=on
  MATLAB Function13 : MATLAB Function  TreatAsAtomicUnit=on
  MATLAB Function14 : MATLAB Function  TreatAsAtomicUnit=on
  MATLAB Function15 : MATLAB Function  TreatAsAtomicUnit=on
  MATLAB Function16 : MATLAB Function  TreatAsAtomicUnit=on
  MATLAB Function17 : MATLAB Function  TreatAsAtomicUnit=on
  MATLAB Function18 : MATLAB Function  TreatAsAtomicUnit=on
  MATLAB Function19 : MATLAB Function  TreatAsAtomicUnit=on
  MATLAB Function2 : MATLAB Function  TreatAsAtomicUnit=on
  MATLAB Function20 : MATLAB Function  TreatAsAtomicUnit=on
  MATLAB Function21 : MATLAB Function  TreatAsAtomicUnit=on
  MATLAB Function22 : MATLAB Function  TreatAsAtomicUnit=on
  MATLAB Function23 : MATLAB Function  TreatAsAtomicUnit=on
  MATLAB Function24 : MATLAB Function  TreatAsAtomicUnit=on
  MATLAB Function25 : MATLAB Function  TreatAsAtomicUnit=on
  MATLAB Function26 : MATLAB Function  TreatAsAtomicUnit=on
  MATLAB Function27 : MATLAB Function  TreatAsAtomicUnit=on
  MATLAB Function28 : MATLAB Function  TreatAsAtomicUnit=on
  MATLAB Function29 : MATLAB Function  TreatAsAtomicUnit=on
  MATLAB Function3 : MATLAB Function  TreatAsAtomicUnit=on
  MATLAB Function30 : MATLAB Function  TreatAsAtomicUnit=on
  MATLAB Function31 : MATLAB Function  TreatAsAtomicUnit=on
  MATLAB Function32 : MATLAB Function  TreatAsAtomicUnit=on
  MATLAB Function33 : MATLAB Function  TreatAsAtomicUnit=on
  MATLAB Function34 : MATLAB Function  TreatAsAtomicUnit=on
  MATLAB Function35 : MATLAB Function  TreatAsAtomicUnit=on
  MATLAB Function36 : MATLAB Function  TreatAsAtomicUnit=on
  MATLAB Function37 : MATLAB Function  TreatAsAtomicUnit=on
  MATLAB Function38 : MATLAB Function  TreatAsAtomicUnit=on
  MATLAB Function39 : MATLAB Function  TreatAsAtomicUnit=on
  MATLAB Function4 : MATLAB Function  TreatAsAtomicUnit=on
  MATLAB Function40 : MATLAB Function  TreatAsAtomicUnit=on
  MATLAB Function41 : MATLAB Function  TreatAsAtomicUnit=on
  MATLAB Function42 : MATLAB Function  TreatAsAtomicUnit=on
  MATLAB Function43 : MATLAB Function  TreatAsAtomicUnit=on
  MATLAB Function44 : MATLAB Function  TreatAsAtomicUnit=on
  MATLAB Function5 : MATLAB Function  TreatAsAtomicUnit=on
  MATLAB Function6 : MATLAB Function  TreatAsAtomicUnit=on
  MATLAB Function7 : MATLAB Function  TreatAsAtomicUnit=on
  MATLAB Function8 : MATLAB Function  TreatAsAtomicUnit=on
  MATLAB Function9 : MATLAB Function  TreatAsAtomicUnit=on
  Mux : Mux  Inputs=50
  Mux2 : Mux  Inputs=2
  SCI_DATA : Outport
  wires:
  Constant1/1 -> Mux/3
  MATLAB Function3/1(TX_DATA) -> MATLAB Function4/1(TX_DATA)
  MATLAB Function4/1(TX_DATA_Hig) -> Mux/5
  Data Store Read21/1 -> MATLAB Function21/1(U1)
  Constant2/1 -> Mux/2
  MATLAB Function25/1(TX_DATA_Hig) -> Mux/11
  MATLAB Function4/2(TX_DATA_Low) -> Mux/6
  MATLAB Function10/1(TX_DATA) -> MATLAB Function27/1(TX_DATA)
  Data Store Read8/1 -> MATLAB Function14/1(RAW_DATA)
  MATLAB Function24/2(TX_DATA_Low) -> Mux/10
  MATLAB Function14/1(TX_DATA) -> MATLAB Function37/1(TX_DATA)
  MATLAB Function23/2(TX_DATA_Low) -> Mux/8
  MATLAB Function26/1(TX_DATA_Hig) -> Mux/13
  MATLAB Function/2(Low) -> MATLAB Function42/1(TX_DATA)
  Data Store Read18/1 -> MATLAB Function1/1(RAW_DATA)
  MATLAB Function18/1(TX_DATA) -> MATLAB Function31/1(TX_DATA)
  MATLAB Function7/1(TX_DATA) -> MATLAB Function36/1(TX_DATA)
  MATLAB Function6/1(TX_DATA) -> MATLAB Function35/1(TX_DATA)
  MATLAB Function16/1(TX_DATA) -> MATLAB Function32/1(TX_DATA)
  MATLAB Function13/1(TX_DATA) -> MATLAB Function30/1(TX_DATA)
  MATLAB Function11/1(TX_DATA) -> MATLAB Function28/1(TX_DATA)
  MATLAB Function1/1(TX_DATA) -> MATLAB Function26/1(TX_DATA)
  1-D Lookup Table1/1 -> MATLAB Function18/1(RAW_DATA)
  Data Store Read5/1 -> MATLAB Function5/1(RAW_DATA)
  MATLAB Function21/1(EFP2) -> MATLAB Function44/1(TX_DATA)
  MATLAB Function15/1(TX_DATA) -> MATLAB Function38/1(TX_DATA)
  Data Store Read19/1 -> MATLAB Function10/1(RAW_DATA)
  MATLAB Function17/1(TX_DATA) -> MATLAB Function33/1(TX_DATA)
  Data Store Read11/1 -> MATLAB Function17/1(RAW_DATA)
  Data Store Read23/1 -> MATLAB Function21/3(U3)
  Data Store Read26/1 -> MATLAB Function21/6(U6)
  Data Store Read25/1 -> MATLAB Function21/5(U5)
  Mux2/1 -> SCI_DATA/1
  Data Store Read24/1 -> MATLAB Function21/4(U4)
  Data Store Read9/1 -> MATLAB Function15/1(RAW_DATA)
  Data Store Read12/1 -> 1-D Lookup Table1/1
  Data Store Read6/1 -> MATLAB Function6/1(RAW_DATA)
  Data Store Read27/1 -> MATLAB Function21/7(U7)
  Data Store Read14/1 -> MATLAB Function11/1(RAW_DATA)
  Data Store Read30/1 -> MATLAB Function21/10(U10)
  MATLAB Function30/2(TX_DATA_Low) -> Mux/22
  Data Store Read2/1 -> MATLAB Function3/1(RAW_DATA)
  MATLAB Function32/1(TX_DATA_Hig) -> Mux/25
  MATLAB Function42/1(TX_DATA_Hig) -> Mux/45
  Data Store Read10/1 -> MATLAB Function16/1(RAW_DATA)
  Data Store Read15/1 -> MATLAB Function12/1(RAW_DATA)
  MATLAB Function44/2(TX_DATA_Low) -> Mux/48
  MATLAB Function36/2(TX_DATA_Low) -> Mux/34
  MATLAB Function43/2(TX_DATA_Low) -> Mux/50
  Data Store Read28/1 -> MATLAB Function21/8(U8)
  MATLAB Function43/1(TX_DATA_Hig) -> Mux/49
  MATLAB Function23/1(TX_DATA_Hig) -> Mux/7
  Constant3/1 -> Mux/1
  MATLAB Function40/2(TX_DATA_Low) -> Mux/42
  MATLAB Function38/2(TX_DATA_Low) -> Mux/38
  MATLAB Function42/2(TX_DATA_Low) -> Mux/46
  MATLAB Function31/1(TX_DATA_Hig) -> Mux/23
  MATLAB Function35/1(TX_DATA_Hig) -> Mux/31
  Constant4/1 -> Mux/4
  MATLAB Function38/1(TX_DATA_Hig) -> Mux/37
  MATLAB Function2/1(TX_DATA) -> MATLAB Function24/1(TX_DATA)
  MATLAB Function39/2(TX_DATA_Low) -> Mux/40
  Data Store Read22/1 -> MATLAB Function21/2(U2)
  MATLAB Function41/1(TX_DATA_Hig) -> Mux/43
  MATLAB Function37/2(TX_DATA_Low) -> Mux/36
  MATLAB Function12/1(TX_DATA) -> MATLAB Function29/1(TX_DATA)
  MATLAB Function35/2(TX_DATA_Low) -> Mux/32
  MATLAB Function37/1(TX_DATA_Hig) -> Mux/35
  MATLAB Function26/2(TX_DATA_Low) -> Mux/14
  MATLAB Function27/2(TX_DATA_Low) -> Mux/16
  MATLAB Function34/2(TX_DATA_Low) -> Mux/30
  MATLAB Function27/1(TX_DATA_Hig) -> Mux/15
  MATLAB Function40/1(TX_DATA_Hig) -> Mux/41
  MATLAB Function33/2(TX_DATA_Low) -> Mux/28
  Data Store Read29/1 -> MATLAB Function21/9(U9)
  MATLAB Function31/2(TX_DATA_Low) -> Mux/24
  MATLAB Function33/1(TX_DATA_Hig) -> Mux/27
  MATLAB Function5/1(TX_DATA) -> MATLAB Function34/1(TX_DATA)
  MATLAB Function28/1(TX_DATA_Hig) -> Mux/17
  Data Store Read3/1 -> MATLAB Function9/1(RAW_DATA)
  MATLAB Function19/1(TX_DATA) -> MATLAB Function39/1(TX_DATA)
  MATLAB Function22/1(TX_DATA) -> Mux2/2
  Data Store Read20/1 -> MATLAB Function20/1(RAW_DATA)
  MATLAB Function/1(High) -> MATLAB Function41/1(TX_DATA)
  MATLAB Function29/2(TX_DATA_Low) -> Mux/20
  MATLAB Function30/1(TX_DATA_Hig) -> Mux/21
  MATLAB Function25/2(TX_DATA_Low) -> Mux/12
  MATLAB Function29/1(TX_DATA_Hig) -> Mux/19
  MATLAB Function28/2(TX_DATA_Low) -> Mux/18
  MATLAB Function9/1(TX_DATA) -> MATLAB Function23/1(TX_DATA)
  MATLAB Function39/1(TX_DATA_Hig) -> Mux/39
  MATLAB Function36/1(TX_DATA_Hig) -> Mux/33
  MATLAB Function32/2(TX_DATA_Low) -> Mux/26
  Data Store Read7/1 -> MATLAB Function7/1(RAW_DATA)
  MATLAB Function41/2(TX_DATA_Low) -> Mux/44
  Data Store Read16/1 -> MATLAB Function13/1(RAW_DATA)
  Data Store Read31/1 -> MATLAB Function21/11(U11)
  Mux/1 -> Mux2/1, MATLAB Function22/1(u)
  MATLAB Function20/1(TX_DATA) -> MATLAB Function40/1(TX_DATA)
  Data Store Read17/1 -> MATLAB Function19/1(RAW_DATA)
  MATLAB Function24/1(TX_DATA_Hig) -> Mux/9
  MATLAB Function34/1(TX_DATA_Hig) -> Mux/29
  MATLAB Function44/1(TX_DATA_Hig) -> Mux/47
  MATLAB Function8/1(TX_DATA) -> MATLAB Function25/1(TX_DATA)
  Data Store Read/1 -> MATLAB Function2/1(RAW_DATA)
  Data Store Read4/1 -> MATLAB Function43/1(TX_DATA)
  Data Store Read1/1 -> MATLAB Function8/1(RAW_DATA)

== system Fuel_Pump_V3_1_20201113_20KHz/Motor_Control/Main Case /AD2S1210 ==
  Data Store Read : DataStoreRead  Commented=on  DataStoreName=SMO_Flag
  Data Store Read1 : DataStoreRead  DataStoreName=Ready_1210
  Data Store Write3 : DataStoreWrite  DataStoreName=n
  If : If
  If Action Subsystem : Subsystem  TreatAsAtomicUnit=on
  SMA_SMO : Subsystem  Commented=on
  Switch : Switch  Commented=on  Criteria=u2 ~= 0
  Terminator : Terminator
  wires:
  Data Store Read1/1 -> If/1
  If/1 -> If Action Subsystem/Action
  If/2 -> Terminator/1
  SMA_SMO/1(n) -> Switch/1
  Data Store Read/1 -> Switch/2
  If Action Subsystem/1(n) -> Data Store Write3/1

== system Fuel_Pump_V3_1_20201113_20KHz/Motor_Control/Main Case /Adjusting Mode ==
  Action Port : ActionPort  ActionPortLabel=case [ 1 ]:

== system Fuel_Pump_V3_1_20201113_20KHz/Motor_Control/Main Case /Clark Transformation ==
  U : Inport
  V : Inport  Port=2
  W : Inport  Port=3
  Add : Sum  Inputs=+--
  Add1 : Sum  Inputs=+-
  Gain : Gain  Gain=0.5
  Gain1 : Gain  Gain=0.5
  Gain2 : Gain  Gain=2/3
  Gain3 : Gain  Gain=2/3*0.86602540
  Alpha : Outport
  Beta : Outport  Port=2
  wires:
  V/1 -> Add1/1, Gain/1
  Gain/1 -> Add/2
  W/1 -> Add1/2, Gain1/1
  Gain1/1 -> Add/3
  U/1 -> Add/1
  Add/1 -> Gain2/1
  Gain2/1 -> Alpha/1
  Add1/1 -> Gain3/1
  Gain3/1 -> Beta/1

== system Fuel_Pump_V3_1_20201113_20KHz/Motor_Control/Main Case /Current Loop Mode ==
  note: Output frequency = Rated_Frequency(666)*rate
  Action Port : ActionPort  ActionPortLabel=case [ 2 ]:
  Constant : Constant  OutDataTypeStr=fixdt(1,32,29)  SampleTime=-1
  Constant1 : Constant  Value=0  OutDataTypeStr=fixdt(1,32,29)  SampleTime=-1
  Data Store Read1 : DataStoreRead  DataStoreName=IF_Frq
  Data Store Write : DataStoreWrite  DataStoreName=Angle
  Data Type Conversion : DataTypeConversion
  Ramp Control : c28xdmclib/Ramp Control  rmp_dly_max=1000  rmp_lo_limit=0  rmp_hi_limit=1
      settings: SourceProductName=Embedded Coder Support Package for Texas Instruments C2000 Processors  SourceProductBaseCode=TIC2000
  Ramp Generator1 : c28xdmclib/Ramp Generator  step_angle_max=666*Ts_20KHz
      settings: SourceProductName=Embedded Coder Support Package for Texas Instruments C2000 Processors  SourceProductBaseCode=TIC2000
  Terminator : Terminator
  wires:
  Constant/1 -> Ramp Generator1/1
  Ramp Generator1/1 -> Data Type Conversion/1
  Constant1/1 -> Ramp Generator1/2
  Ramp Control/2 -> Terminator/1
  Ramp Control/1 -> Ramp Generator1/3
  Data Type Conversion/1 -> Data Store Write/1
  Data Store Read1/1 -> Ramp Control/1

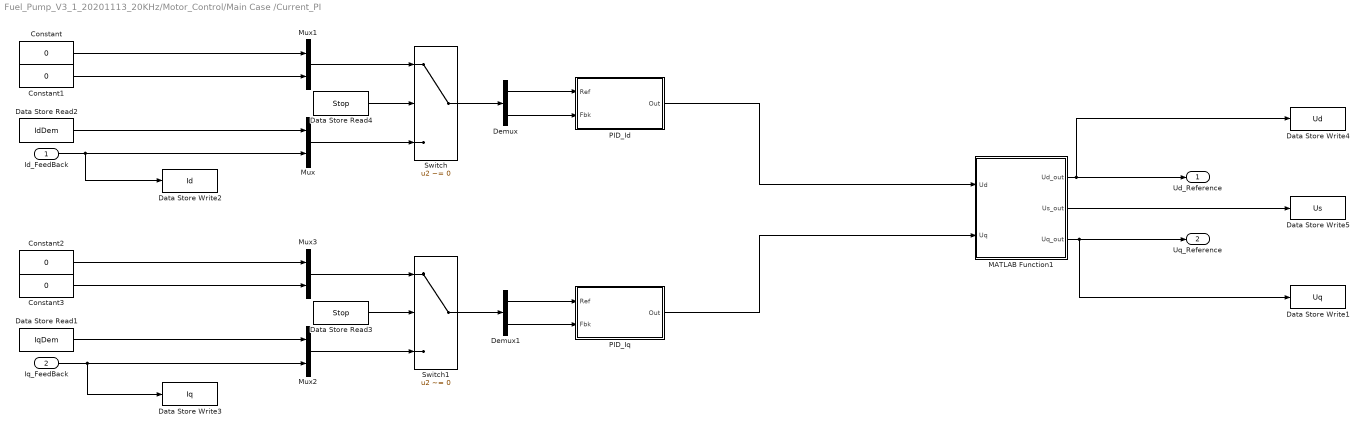
== system Fuel_Pump_V3_1_20201113_20KHz/Motor_Control/Main Case /Current_PI ==
  Id_FeedBack : Inport
  Iq_FeedBack : Inport  Port=2
  Constant{,1..3} (4 alike) : Constant  Value=0  OutDataTypeStr=single  SampleTime=-1
  Data Store Read1 : DataStoreRead  DataStoreName=IqDem
  Data Store Read2 : DataStoreRead  DataStoreName=IdDem
  Data Store Read3 : DataStoreRead  DataStoreName=Stop
  Data Store Read4 : DataStoreRead  DataStoreName=Stop
  Data Store Write1 : DataStoreWrite  DataStoreName=Uq
  Data Store Write2 : DataStoreWrite  DataStoreName=Id
  Data Store Write3 : DataStoreWrite  DataStoreName=Iq
  Data Store Write4 : DataStoreWrite  DataStoreName=Ud
  Data Store Write5 : DataStoreWrite  DataStoreName=Us
  Demux : Demux  Outputs=2
  Demux1 : Demux  Outputs=2
  MATLAB Function1 : MATLAB Function  TreatAsAtomicUnit=on
  Mux{,1..3} (4 alike) : Mux  Inputs=2
  "PID_Id " : Subsystem
  PID_Iq : Subsystem
  Switch : Switch  Criteria=u2 ~= 0
  Switch1 : Switch  Criteria=u2 ~= 0
  Ud_Reference : Outport
  Uq_Reference : Outport  Port=2
  wires:
  "PID_Id "/1(Out) -> MATLAB Function1/1(Ud)
  PID_Iq/1(Out) -> MATLAB Function1/2(Uq)
  Demux/1 -> "PID_Id "/1(Ref)
  Data Store Read4/1 -> Switch/2
  Constant/1 -> Mux1/1
  Mux1/1 -> Switch/1
  Demux/2 -> "PID_Id "/2(Fbk)
  Mux/1 -> Switch/3
  Constant1/1 -> Mux1/2
  Switch/1 -> Demux/1
  Data Store Read2/1 -> Mux/1
  Demux1/2 -> PID_Iq/2(Fbk)
  Data Store Read1/1 -> Mux2/1
  Constant2/1 -> Mux3/1
  Switch1/1 -> Demux1/1
  Constant3/1 -> Mux3/2
  Mux2/1 -> Switch1/3
  Data Store Read3/1 -> Switch1/2
  Demux1/1 -> PID_Iq/1(Ref)
  Mux3/1 -> Switch1/1
  Iq_FeedBack/1 -> Data Store Write3/1, Mux2/2
  Id_FeedBack/1 -> Mux/2, Data Store Write2/1
  MATLAB Function1/3(Uq_out) -> Uq_Reference/1, Data Store Write1/1
  MATLAB Function1/1(Ud_out) -> Data Store Write4/1, Ud_Reference/1
  MATLAB Function1/2(Us_out) -> Data Store Write5/1

== system Fuel_Pump_V3_1_20201113_20KHz/Motor_Control/Main Case /Data Buffer  ==
  Data Store Read : DataStoreRead  DataStoreName=Id
  Data Store Read1 : DataStoreRead  DataStoreName=IqDem
  Data Store Read2 : DataStoreRead  DataStoreName=IdDem
  Data Store Read3 : DataStoreRead  DataStoreName=Iq
  Data Store Read4 : DataStoreRead  DataStoreName=AD_Angle
  Data Store Read5 : DataStoreRead  DataStoreName=SMO_Theta
  MATLAB Function1 : MATLAB Function  TreatAsAtomicUnit=on
  wires:
  Data Store Read2/1 -> MATLAB Function1/5(IdDem)
  Data Store Read1/1 -> MATLAB Function1/3(IqDem)
  Data Store Read/1 -> MATLAB Function1/6(Id)
  Data Store Read3/1 -> MATLAB Function1/4(Iq)
  Data Store Read4/1 -> MATLAB Function1/2(ThetaAD2S)
  Data Store Read5/1 -> MATLAB Function1/1(ThetaSMO)

== system Fuel_Pump_V3_1_20201113_20KHz/Motor_Control/Main Case /Error ==
  Action Port : ActionPort  ActionPortLabel=default:
  Constant : Constant  Value=0  OutDataTypeStr=single  SampleTime=-1
  Constant1 : Constant  OutDataTypeStr=uint16  SampleTime=-1
  Data Store Write : DataStoreWrite  DataStoreName=Angle
  Data Store Write1 : DataStoreWrite  DataStoreName=Stop
  wires:
  Constant/1 -> Data Store Write/1
  Constant1/1 -> Data Store Write1/1

== system Fuel_Pump_V3_1_20201113_20KHz/Motor_Control/Main Case /If Action Subsystem ==
  Action Port : ActionPort  ActionPortLabel=if(u1 == 1)
  Constant : Constant  Value=0  OutDataTypeStr=single  SampleTime=-1
  Constant1 : Constant  Value=0  OutDataTypeStr=single  SampleTime=-1
  Constant2 : Constant  Value=0  OutDataTypeStr=single  SampleTime=-1
  Data Store Write1 : DataStoreWrite  DataStoreName=uiId
  Data Store Write2 : DataStoreWrite  DataStoreName=uiIq
  Data Store Write3 : DataStoreWrite  DataStoreName=uin
  wires:
  Constant/1 -> Data Store Write1/1
  Constant1/1 -> Data Store Write2/1
  Constant2/1 -> Data Store Write3/1

== system Fuel_Pump_V3_1_20201113_20KHz/Motor_Control/Main Case /Park Transformation ==
  Alpha : Inport
  Beta : Inport  Port=2
  theta : Inport  Port=3
  Add : Sum
  Add1 : Sum  Inputs=+-
  Gain : Gain  Gain=2*pi  OutDataTypeStr=single
  Product{,1..3} (4 alike) : Product
  Sin : Trigonometry  OutputSignalType=real
  Sin1 : Trigonometry  Operator=cos  OutputSignalType=real
  D : Outport
  Q : Outport  Port=2
  wires:
  Product/1 -> Add/1
  Sin/1 -> Product3/2, Product1/2
  Product1/1 -> Add/2
  Add1/1 -> Q/1
  Sin1/1 -> Product2/2, Product/2
  Product2/1 -> Add1/1
  Alpha/1 -> Product3/1, Product/1
  Beta/1 -> Product2/1, Product1/1
  theta/1 -> Gain/1
  Product3/1 -> Add1/2
  Add/1 -> D/1
  Gain/1 -> Sin/1, Sin1/1

== system Fuel_Pump_V3_1_20201113_20KHz/Motor_Control/Main Case /Position Loop Mode ==
  Action Port : ActionPort  ActionPortLabel=case [ 3 ]:
  Data Store Read : DataStoreRead  DataStoreName=AD_Angle
  Data Store Write : DataStoreWrite  DataStoreName=Angle
  If Action Subsystem : Subsystem  TreatAsAtomicUnit=on
  MATLAB Function : MATLAB Function  TreatAsAtomicUnit=on
  wires:
  MATLAB Function/1(SPEED_PI()) -> If Action Subsystem/Trigger
  Data Store Read/1 -> Data Store Write/1

== system Fuel_Pump_V3_1_20201113_20KHz/Motor_Control/Main Case /SVPWM ==
  Ud_Reference : Inport
  Uq_Reference : Inport  Port=2
  Angle : Inport  Port=3
  Constant : Constant  Value=TPBRD_HALF  OutDataTypeStr=single  SampleTime=-1
  Data Store Write : DataStoreWrite  DataStoreName=V_alpha
  Data Store Write1 : DataStoreWrite  DataStoreName=V_beta
  Gain : Gain  Gain=TPBRD_HALF  OutDataTypeStr=single  ParamDataTypeStr=Inherit: Same as input
  Gain1 : Gain  Gain=1/MotorPara_Base_V
  Inverse Park Transformation : Subsystem
  MATLAB Function : MATLAB Function  TreatAsAtomicUnit=on
  Mux : Mux  Inputs=3
  Sum1 : Sum  Inputs=|-+  OutDataTypeStr=uint16
  COMPARE : Outport
  wires:
  Angle/1 -> Inverse Park Transformation/3(theta)
  Mux/1 -> Gain1/1
  Uq_Reference/1 -> Inverse Park Transformation/2(Q)
  Constant/1 -> Sum1/2
  Gain/1 -> Sum1/1
  Sum1/1 -> COMPARE/1
  Ud_Reference/1 -> Inverse Park Transformation/1(D)
  Inverse Park Transformation/1(Alpha) -> Data Store Write/1, MATLAB Function/1(alpha)
  MATLAB Function/1(ta) -> Mux/1
  MATLAB Function/2(tb) -> Mux/2
  MATLAB Function/3(tc) -> Mux/3
  Gain1/1 -> Gain/1
  Inverse Park Transformation/2(Beta) -> Data Store Write1/1, MATLAB Function/2(beta)

== system Fuel_Pump_V3_1_20201113_20KHz/Motor_Control/Main Case /Speed Loop Mode ==
  Action Port : ActionPort  ActionPortLabel=case [ 5 ]:
  Data Store Read : DataStoreRead  DataStoreName=AD_Angle
  Data Store Read1 : DataStoreRead  DataStoreName=SMO_Theta
  Data Store Read2 : DataStoreRead  DataStoreName=SMO_Flag
  Data Store Write : DataStoreWrite  DataStoreName=Angle
  If Action Subsystem : Subsystem  TreatAsAtomicUnit=on
  MATLAB Function : MATLAB Function  TreatAsAtomicUnit=on
  MATLAB Function1 : MATLAB Function  TreatAsAtomicUnit=on
  wires:
  MATLAB Function/1(SPEED_PI()) -> If Action Subsystem/Trigger
  Data Store Read/1 -> MATLAB Function1/1(Theta_1210)
  Data Store Read1/1 -> MATLAB Function1/3(Theta_SMO)
  Data Store Read2/1 -> MATLAB Function1/2(SMO_Flag)
  MATLAB Function1/1(Theta) -> Data Store Write/1

== system Fuel_Pump_V3_1_20201113_20KHz/Motor_Control/Main Case /Stop ==
  Action Port : ActionPort  ActionPortLabel=case [ 0 ]:
  Constant : Constant  Value=0  OutDataTypeStr=single  SampleTime=-1
  Constant1 : Constant  OutDataTypeStr=uint16  SampleTime=-1
  Data Store Write : DataStoreWrite  DataStoreName=Angle
  Data Store Write1 : DataStoreWrite  DataStoreName=Stop
  wires:
  Constant1/1 -> Data Store Write1/1
  Constant/1 -> Data Store Write/1

== system Fuel_Pump_V3_1_20201113_20KHz/Motor_Control/Main Case /VVF Mode ==
  note: Output frequency = Rated_Frequency(800)*rate
  Action Port : ActionPort  ActionPortLabel=case [ 4 ]:
  Constant : Constant  OutDataTypeStr=fixdt(1,32,29)  SampleTime=-1
  Constant1 : Constant  Value=0  OutDataTypeStr=fixdt(1,32,29)  SampleTime=-1
  Data Store Write : DataStoreWrite  DataStoreName=Angle
  Data Type Conversion : DataTypeConversion
  Ramp Control : c28xdmclib/Ramp Control  rmp_dly_max=1  rmp_lo_limit=0  rmp_hi_limit=1
      settings: SourceProductName=Embedded Coder Support Package for Texas Instruments C2000 Processors  SourceProductBaseCode=TIC2000
  Ramp Generator1 : c28xdmclib/Ramp Generator  step_angle_max=666*Ts_20KHz
      settings: SourceProductName=Embedded Coder Support Package for Texas Instruments C2000 Processors  SourceProductBaseCode=TIC2000
  Rate : DataStoreRead  DataStoreName=VVF_Frq
  Terminator : Terminator
  wires:
  Data Type Conversion/1 -> Data Store Write/1
  Constant1/1 -> Ramp Generator1/2
  Constant/1 -> Ramp Generator1/1
  Ramp Control/1 -> Ramp Generator1/3
  Ramp Generator1/1 -> Data Type Conversion/1
  Ramp Control/2 -> Terminator/1
  Rate/1 -> Ramp Control/1
